simulink model "LookUpTableTest"  (R2016b)
settings: Solver=ode5  StartTime=0.0  StopTime=20  FixedStep=.001  RelTol=1e-3
values from neighbouring files (symbols this model uses):
  data =     [EstimatedParameters.mat]    (also in initialization.mat)
  LookUpTablesDelayBetweenChannels = 0    [init.m]    (also in initialization.mat)
  LookUpTablesStartDelay = 0    [init.m]    (also in initialization.mat)
  TimeRPY = [0 0.05 0.1 0.15 0.2 0.25 0.3 0.35 0.4 0.45 0.5 0.55 ... (215 elements, 1x215)]    [EstimatedParameters.mat]    (also in initialization.mat)
libraries: cstblocks x1
settings Model: Creator=aghersin  LastModifiedBy=aghersin

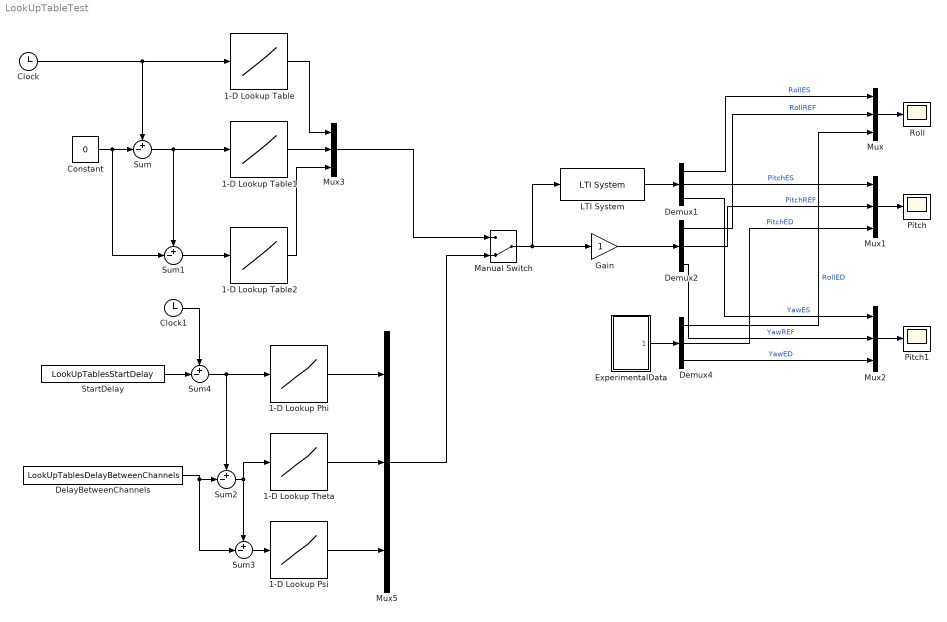
== system LookUpTableTest ==
  1-D Lookup Phi : Lookup_n-D  NumberOfTableDimensions=1  BreakpointsForDimension1=[0:length(TimeRPY)-1+20+20]*data.Ts  Table=[zeros(20,1);data.InputData(:,1);zeros(20,1)]  InterpMethod=Cubic spline  ExtrapMethod=Cubic spline  InternalRulePriority=Speed  RndMeth=Simplest  InputSameDT=on
  1-D Lookup Psi : Lookup_n-D  NumberOfTableDimensions=1  BreakpointsForDimension1=[0:length(TimeRPY)-1+20+20]*data.Ts  Table=[data.InputData(1,3)*ones(20,1);data.InputData(:,3);data.InputData(end,3)*ones(20,1)]  InterpMethod=Cubic spline  ExtrapMethod=Cubic spline  InternalRulePriority=Speed  RndMeth=Simplest  InputSameDT=on
  1-D Lookup Table : Lookup_n-D  NumberOfTableDimensions=1  BreakpointsForDimension1=[0:length(TimeRPY)-1+20+20]*data.Ts  Table=[zeros(20,1);data.InputData(:,1);zeros(20,1)]  InterpMethod=Cubic spline  ExtrapMethod=Cubic spline  InternalRulePriority=Speed  RndMeth=Simplest  InputSameDT=on
  1-D Lookup Table1 : Lookup_n-D  NumberOfTableDimensions=1  BreakpointsForDimension1=[0:length(TimeRPY)-1+20+20]*data.Ts  Table=[zeros(20,1);data.InputData(:,2);zeros(20,1)]  InterpMethod=Cubic spline  ExtrapMethod=Cubic spline  InternalRulePriority=Speed  RndMeth=Simplest  InputSameDT=on
  1-D Lookup Table2 : Lookup_n-D  NumberOfTableDimensions=1  BreakpointsForDimension1=[0:length(TimeRPY)-1+20+20]*data.Ts  Table=[data.InputData(1,3)*ones(20,1);data.InputData(:,3);data.InputData(end,3)*ones(20,1)]  InterpMethod=Cubic spline  ExtrapMethod=Cubic spline  InternalRulePriority=Speed  RndMeth=Simplest  InputSameDT=on
  1-D Lookup Theta : Lookup_n-D  NumberOfTableDimensions=1  BreakpointsForDimension1=[0:length(TimeRPY)-1+20+20]*data.Ts  Table=[zeros(20,1);data.InputData(:,2);zeros(20,1)]  InterpMethod=Cubic spline  ExtrapMethod=Cubic spline  InternalRulePriority=Speed  RndMeth=Simplest  InputSameDT=on
  Clock : Clock
  Clock1 : Clock
  Constant : Constant  Value=0
  DelayBetweenChannels : Constant  Value=LookUpTablesDelayBetweenChannels
  Demux1 : Demux  Outputs=3
  Demux2 : Demux  Outputs=3
  Demux4 : Demux  Outputs=3
  ExperimentalData : Subsystem
  Gain : Gain
  LTI System : cstblocks/LTI System  sys=RPYEstSysss  IC=[]
  Manual Switch : ManualSwitch  CurrentSetting=0
  Mux{,1..3,5} (5 alike) : Mux  Inputs=3
  Pitch : Scope
  Pitch1 : Scope
  Roll : Scope
  StartDelay : Constant  Value=LookUpTablesStartDelay
  Sum{,1..4} (5 alike) : Sum  Inputs=+-|
  wires:
  Clock/1 -> 1-D Lookup Table/1, Sum/1
  Sum/1 -> 1-D Lookup Table1/1, Sum1/1
  Sum1/1 -> 1-D Lookup Table2/1
  Constant/1 -> Sum1/2, Sum/2
  Demux1/2 -> Mux1/1  "PitchES"
  Mux/1 -> Roll/1
  Demux1/3 -> Mux2/1  "YawES"
  Mux2/1 -> Pitch1/1
  Demux1/1 -> Mux/1  "RollES"
  Mux1/1 -> Pitch/1
  Demux2/2 -> Mux1/2  "PitchREF"
  Demux2/3 -> Mux2/2  "YawREF"
  Mux3/1 -> Manual Switch/1
  Demux2/1 -> Mux/2  "RollREF"
  Demux4/1 -> Mux/3  "RollED"
  Demux4/2 -> Mux1/3  "PitchED"
  Demux4/3 -> Mux2/3  "YawED"
  ExperimentalData/1(RollPitchYaw) -> Demux4/1
  Gain/1 -> Demux2/1
  LTI System/1 -> Demux1/1
  1-D Lookup Table/1 -> Mux3/1
  1-D Lookup Table1/1 -> Mux3/2
  1-D Lookup Table2/1 -> Mux3/3
  DelayBetweenChannels/1 -> Sum3/2, Sum2/2
  Sum3/1 -> 1-D Lookup Psi/1
  Sum2/1 -> 1-D Lookup Theta/1, Sum3/1
  Clock1/1 -> Sum4/1
  1-D Lookup Psi/1 -> Mux5/3
  Mux5/1 -> Manual Switch/2
  StartDelay/1 -> Sum4/2
  Sum4/1 -> Sum2/1, 1-D Lookup Phi/1
  Manual Switch/1 -> Gain/1, LTI System/1
  1-D Lookup Phi/1 -> Mux5/1
  1-D Lookup Theta/1 -> Mux5/2

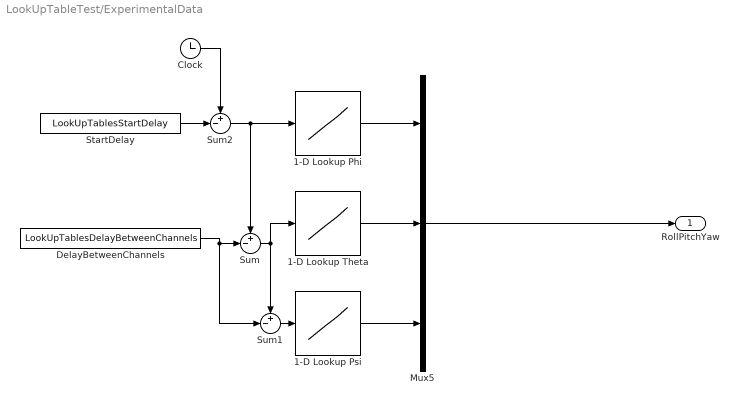
== system LookUpTableTest/ExperimentalData ==
  1-D Lookup Phi : Lookup_n-D  NumberOfTableDimensions=1  BreakpointsForDimension1=[0:length(TimeRPY)-1+20+20]*data.Ts  Table=[zeros(20,1);data.OutputData(:,1);zeros(20,1)]  InterpMethod=Cubic spline  ExtrapMethod=Cubic spline  InternalRulePriority=Speed  RndMeth=Simplest  InputSameDT=on
  1-D Lookup Psi : Lookup_n-D  NumberOfTableDimensions=1  BreakpointsForDimension1=[0:length(TimeRPY)-1+20+20]*data.Ts  Table=[data.InputData(1,3)*ones(20,1);data.OutputData(:,3);data.InputData(end,3)*ones(20,1)]  InterpMethod=Cubic spline  ExtrapMethod=Cubic spline  InternalRulePriority=Speed  RndMeth=Simplest  InputSameDT=on
  1-D Lookup Theta : Lookup_n-D  NumberOfTableDimensions=1  BreakpointsForDimension1=[0:length(TimeRPY)-1+20+20]*data.Ts  Table=[zeros(20,1);data.OutputData(:,2);zeros(20,1)]  InterpMethod=Cubic spline  ExtrapMethod=Cubic spline  InternalRulePriority=Speed  RndMeth=Simplest  InputSameDT=on
  Clock : Clock
  DelayBetweenChannels : Constant  Value=LookUpTablesDelayBetweenChannels
  Mux5 : Mux  Inputs=3
  StartDelay : Constant  Value=LookUpTablesStartDelay
  Sum : Sum  Inputs=+-|
  Sum1 : Sum  Inputs=+-|
  Sum2 : Sum  Inputs=+-|
  RollPitchYaw : Outport
  wires:
  Mux5/1 -> RollPitchYaw/1
  1-D Lookup Psi/1 -> Mux5/3
  DelayBetweenChannels/1 -> Sum1/2, Sum/2
  Sum1/1 -> 1-D Lookup Psi/1
  Sum/1 -> 1-D Lookup Theta/1, Sum1/1
  Clock/1 -> Sum2/1
  StartDelay/1 -> Sum2/2
  Sum2/1 -> 1-D Lookup Phi/1, Sum/1
  1-D Lookup Theta/1 -> Mux5/2
  1-D Lookup Phi/1 -> Mux5/1
